simulink model "Lab3_Soh_Nguyen_Kho_AbdulKadir_simulink"  (R2021a)
settings: Solver=VariableStepAuto  StartTime=0.0  StopTime=20  MaxStep=0.001  RelTol=1e-3
libraries: cstblocks x2
settings Model: Creator=kkqi_  LastModifiedBy=kkqi_

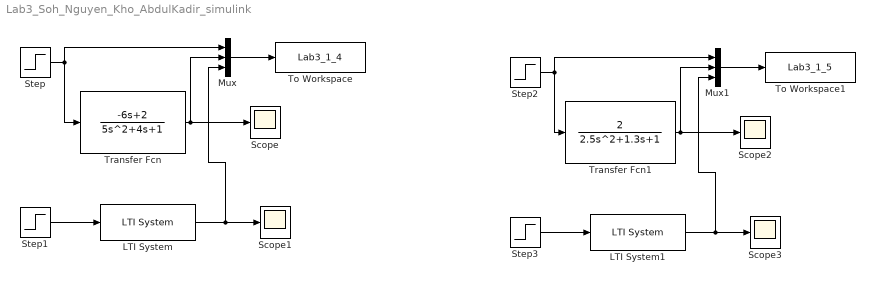
== system Lab3_Soh_Nguyen_Kho_AbdulKadir_simulink ==
  LTI System : cstblocks/LTI System  sys=tf(2,[5 1],'ioDelay',2)  IC=[]
  LTI System1 : cstblocks/LTI System  sys=tf(2,[2 1],'ioDelay',.2)  IC=[]
  Mux : Mux  Inputs=3
  Mux1 : Mux  Inputs=3
  Scope{,1..3} (4 alike) : Scope
  Step{,1..3} (4 alike) : Step  Time=2  SampleTime=0
  To Workspace : ToWorkspace  VariableName=Lab3_1_4  SampleTime=-1
  To Workspace1 : ToWorkspace  VariableName=Lab3_1_5  SampleTime=-1
  Transfer Fcn : TransferFcn  Numerator=[-6 2]  Denominator=[5 4 1]
  Transfer Fcn1 : TransferFcn  Numerator=[2]  Denominator=[2.5 1.3 1]
  wires:
  Step/1 -> Transfer Fcn/1, Mux/1
  Transfer Fcn/1 -> Mux/2, Scope/1
  Mux/1 -> To Workspace/1
  Step1/1 -> LTI System/1
  LTI System/1 -> Mux/3, Scope1/1
  LTI System1/1 -> Mux1/3, Scope3/1
  Step3/1 -> LTI System1/1
  Mux1/1 -> To Workspace1/1
  Transfer Fcn1/1 -> Mux1/2, Scope2/1
  Step2/1 -> Transfer Fcn1/1, Mux1/1
